simulink model "bObserver"  (R2020a)
settings: Solver=VariableStepAuto  StartTime=0.0  StopTime=1.5  FixedStep=0.0005  EnableMultiTasking=on
InitFcn:
  | kp=0.01;
  | ki=0.01;
  | 
  | k=2;
  | em=100000000;
  | GE=1/em;
  | GU=k*ki/GE;
  | GCE=k*kp/GU;
model workspace (MAT data in the model file):
  time = 0.8
values from neighbouring files (symbols this model uses):
  A1 = obj.boostConverter.A1    [BoostController.m]    (also in BoostConverter.m = [-obj.R/obj.L 0;0 -1/(obj.Ro*obj.C)]; BuckBoostConverter.m = [-obj.R/obj.L 0;0 -1/(obj.Ro*obj.C)]; obsmc.m = Asigma{1,1}; workspace_atual.mat = [-16.4  0; 0  -3.50877192982])
  A2 = obj.boostConverter.A2    [BoostController.m]    (also in BoostConverter.m = [-obj.R/obj.L -1/obj.L;1/obj.C -1/(obj.Ro*obj.C)]; BuckBoostConverter.m = [-obj.R/obj.L 1/obj.L;-1/obj.C -1/(obj.Ro*obj.C)]; obsmc.m = Asigma{1,2}; workspace_atual.mat = [-16.4  -200; 350.877192982  -3.50877192982])
  AlarmDeadTime = 0.50    (= 0.5)    [BoostFaultSimulation.m]    (also in workspace_atual.mat; workspace_certo.mat)
  B1 = obj.boostConverter.B1    [BoostController.m]    (also in BoostConverter.m = [1/obj.L;0]; BuckBoostConverter.m = [1/obj.L;0]; obsmc.m = Bsigma{1,1}; workspace_atual.mat = [200 0])
  B1f = [200 0]    [workspace_atual.mat]    (also in workspace_certo.mat)
  B2 = obj.boostConverter.B2    [BoostController.m]    (also in BoostConverter.m = obj.B1; obsmc.m = Bsigma{1,2}; workspace_atual.mat = [200 0]; workspace_certo.mat = [200 0])
  B2f = [200 0]    [workspace_atual.mat]    (also in workspace_certo.mat)
  boost_Amatrices = cat(3,obj.A1,obj.A2)    [BoostConverter.m]    (also in BuckBoostConverter.m; boostResults2Latex.m = boost.A_matrices(); workspace_atual.mat = [-16.4 0 0 -3.50877192982 -16.4 350.877192982 -200 -3.508771; workspace_certo.mat = [-16.4 0 0 -3.50877192982 -16.4 350.877192982 -200 -3.508771)
  boost_parameters = [obj.Ro,obj.R,obj.L,obj.C,obj.u]'    [BoostConverter.m]    (also in BuckBoostConverter.m; boostResults2Latex.m = boost.parameters(); workspace_atual.mat = [100 0.082 0.005 0.00285 190]; workspace_certo.mat = [100 0.082 0.005 0.00285 190])
  C = 1e-3    (= 0.001)    [boostResults2Latex.m]
  CiL = [0 1]    [workspace_atual.mat]    (also in workspace_certo.mat)
  Cmatrix = [1  0; 0  1]    [workspace_atual.mat]    (also in workspace_certo.mat)
  CVc = [1 0]    [workspace_atual.mat]    (also in workspace_certo.mat)
  D1 = [1  0; 0  1]    [workspace_atual.mat]    (also in workspace_certo.mat)
  F_11 = -16.4    [workspace_atual.mat]    (also in workspace_certo.mat)
  F_12 = -4812476.87956    [workspace_atual.mat]    (also in workspace_certo.mat)
  F_21 = -3.50877192982    [workspace_atual.mat]    (also in workspace_certo.mat)
  F_22 = -2.00703596657    [workspace_atual.mat]    (also in workspace_certo.mat)
  FaultClass = 0    [BoostFaultSimulation.m]    (also in workspace_atual.mat = 1; workspace_certo.mat = 1)
  H_1 = 13715.5123667    [workspace_atual.mat]    (also in workspace_certo.mat)
  iLFaultSwitch = 0    [BoostFaultSimulation.m]    (also in workspace_atual.mat; workspace_certo.mat)
  iLFaultTime = 1.70    (= 1.7)    [BoostFaultSimulation.m]    (also in workspace_atual.mat; workspace_certo.mat)
  iLGainFaultFactor = 15    [BoostFaultSimulation.m]    (also in workspace_atual.mat; workspace_certo.mat)
  iLNoiseFaultSwitch = 0    [BoostFaultSimulation.m]    (also in workspace_atual.mat; workspace_certo.mat)
  iLNoiseTime = 1.70    (= 1.7)    [BoostFaultSimulation.m]    (also in workspace_atual.mat; workspace_certo.mat)
  Jth = 2000    [workspace_atual.mat]    (also in workspace_certo.mat)
  L = 1e-3    (= 0.001)    [boostResults2Latex.m]    (also in obsmc.m = sdpvar(3,1,'full'))
  L_11 = -176809.798019    [workspace_atual.mat]    (also in workspace_certo.mat)
  L_12 = -66005538231.6    [workspace_atual.mat]    (also in workspace_certo.mat)
  L_21 = 0.0967961040176    [workspace_atual.mat]    (also in workspace_certo.mat)
  L_22 = 350.985265141    [workspace_atual.mat]    (also in workspace_certo.mat)
  LoadAddSignalSwitch = 1    [BoostFaultSimulation.m]    (also in workspace_atual.mat; workspace_certo.mat)
  LoadAddSwitch = 0    [BoostFaultSimulation.m]    (also in workspace_atual.mat; workspace_certo.mat)
  LoadAddTime = 0.90    (= 0.9)    [BoostFaultSimulation.m]    (also in workspace_atual.mat; workspace_certo.mat)
  LoadRemoveSignalSwitch = 1    [BoostFaultSimulation.m]    (also in workspace_atual.mat; workspace_certo.mat)
  LoadRemoveSwitch = 0    [BoostFaultSimulation.m]    (also in workspace_atual.mat; workspace_certo.mat)
  LoadRemoveTime = 0.90    (= 0.9)    [BoostFaultSimulation.m]    (also in workspace_atual.mat; workspace_certo.mat)
  LobsiL = [1737913.15707 66180.0912281]    [workspace_atual.mat]    (also in workspace_certo.mat)
  LobsVc = [61200 1]    [workspace_atual.mat]    (also in workspace_certo.mat)
  ObsEp = 70    [workspace_atual.mat]    (also in workspace_certo.mat)
  P = value(P)    [BoostController.m]    (also in boostResults2Latex.m = boost.calculateP(); obsmc.m = blkdiag(1/deltaAtilde(1,2),-1/deltaAtilde(2,1),1); workspace_atual.mat = [0.00235275094895  5.25738510027e-05; 5.25738510027e-05  0.0; workspace_certo.mat = [0.00235275094893  5.25738512446e-05; 5.25738512446e-05  0.0)
  Q_1 = [13715.5123667  1; 1  0]    [workspace_atual.mat]    (also in workspace_certo.mat)
  Q_2 = [1  0; 0.00750867981628  1]    [workspace_atual.mat]    (also in workspace_certo.mat)
  R = 0.1    [boostResults2Latex.m]    (also in workspace_atual.mat = 0.082; workspace_certo.mat = 0.082)
  ReconfigSwitch = 0    [BoostFaultSimulation.m]    (also in workspace_atual.mat; workspace_certo.mat)
  ReconfigTime = 1.707    [BoostFaultSimulation.m]    (also in workspace_atual.mat; workspace_certo.mat)
  rho = 5    [workspace_atual.mat]    (also in workspace_certo.mat)
  RMSfrequency = 47.61    [BoostFaultSimulation.m]    (also in workspace_atual.mat; workspace_certo.mat)
  Ro = 100    [BoostFaultSimulation.m]    (also in boostResults2Latex.m = 10; workspace_atual.mat; workspace_certo.mat)
  Smep = 80    [workspace_atual.mat]    (also in workspace_certo.mat)
  SourceAddSignalSwitch = 1    [BoostFaultSimulation.m]    (also in workspace_atual.mat; workspace_certo.mat)
  SourceAddSwitch = 0    [BoostFaultSimulation.m]    (also in workspace_atual.mat; workspace_certo.mat)
  SourceAddTime = 0.90    (= 0.9)    [BoostFaultSimulation.m]    (also in workspace_atual.mat; workspace_certo.mat)
  SourceAddVoltage = obj.SourceAddFactor*obj.u    [BoostFaultSimulation.m]    (also in workspace_atual.mat = 19; workspace_certo.mat = 19)
  SourceRemoveSignalSwitch = 1    [BoostFaultSimulation.m]    (also in workspace_atual.mat; workspace_certo.mat)
  SourceRemoveSwitch = 0    [BoostFaultSimulation.m]    (also in workspace_atual.mat; workspace_certo.mat)
  SourceRemoveTime = 0.90    (= 0.9)    [BoostFaultSimulation.m]    (also in workspace_atual.mat; workspace_certo.mat)
  SourceRemoveVoltage = obj.SourceRemoveFactor*obj.u    [BoostFaultSimulation.m]    (also in workspace_atual.mat = 19; workspace_certo.mat = 19)
  T_1 = [1 -13715.5123667]    [workspace_atual.mat]    (also in workspace_certo.mat)
  T_2 = [-0.00750867981628 1]    [workspace_atual.mat]    (also in workspace_certo.mat)
  ueq = 0.5    [workspace_atual.mat]    (also in workspace_certo.mat)
  uf = 190    [workspace_atual.mat]    (also in workspace_certo.mat)
  VcFaultSwitch = 0    [BoostFaultSimulation.m]    (also in workspace_atual.mat; workspace_certo.mat)
  VcFaultTime = 1.70    (= 1.7)    [BoostFaultSimulation.m]    (also in workspace_atual.mat; workspace_certo.mat)
  VcGainFaultFactor = 15    [BoostFaultSimulation.m]    (also in workspace_atual.mat; workspace_certo.mat)
  VcNoiseFaultSwitch = 0    [BoostFaultSimulation.m]    (also in workspace_atual.mat; workspace_certo.mat)
  VcNoiseTime = 1.70    (= 1.7)    [BoostFaultSimulation.m]    (also in workspace_atual.mat; workspace_certo.mat)
  ve = 380    [BoostFaultSimulation.m]    (also in boostResults2Latex.m = 100; workspace_atual.mat; workspace_certo.mat)
  x_e = [ie;ve]    [BoostConverter.m]    (also in BuckBoostConverter.m)
  xe = obj.boostConverter.equilibriumstate(ve)    [BoostController.m]    (also in workspace_atual.mat = [7.62509288104 380]; workspace_certo.mat = [7.62509288104 380])
undefined symbols (not defined in the file or in its folder): Atilde1, Atilde2, B1u, Ctilde1, Dtilde1, Dtilde2, F, F1, G, G1, MAXnet, MINnet
libraries: neural x36, powerlib x34, dspstat3 x11, PhdLibrary x10, simulink x7, dspmtrx3 x6, powerlib_meascontrol x4, dspmathops x4
(part 4 of 6)

== system bObserver/Slding Mode/ErrorGenerator/If Action Subsystem ==
  e_y : Inport
  Action Port : ActionPort  ActionPortLabel=if(u1 ~= 0)
  Matrix Multiply : Product  Multiplication=Matrix(*)
  Matrix Multiply1 : Product
  Matrizes A1 : Constant  Value=rho
  Matrizes A2 : Constant  Value=F
  Normalization : dspmathops/Normalization  NormType=2-norm  Bias=1e-10  NormOver=Each column  Dimension=1  roundingMode=Floor  overflowMode=off  accumDataTypeStr=Inherit: Same as product output  accumLastDataTypeStr=Inherit: Same as product output  outputDataTypeStr=Inherit: Same as product output  outputMin=[]  outputMax=[]  outputLastDataTypeStr=Inherit: Same as product output
  v : Outport
  wires:
  Matrix Multiply/1 -> Normalization/1
  Matrizes A2/1 -> Matrix Multiply/1
  Normalization/1 -> Matrix Multiply1/2
  e_y/1 -> Matrix Multiply/2
  Matrizes A1/1 -> Matrix Multiply1/1
  Matrix Multiply1/1 -> v/1

== system bObserver/Slding Mode/ErrorGenerator/If Action Subsystem1 ==
  e_y : Inport
  Action Port : ActionPort  ActionPortLabel=else
  v : Outport
  wires:
  e_y/1 -> v/1

== system bObserver/Slding Mode/Fault Identification Neural Netowrk/Pattern Recognition Neural Network1 ==
  Input : Inport  PortDimensions=3
      mask Display: e = 0.06;c1 = [120 230 180]/255;c2 = ([120 230 180]+0)/(256+128);c3 = ([120 230 180]+128)/(256+128);patch([0 1 1 0],[0 0 1 1],c1);patch([0 1 1 1-e 1-e 0+e],[0 0 1 1-e 0+e 0+e],c2);patch([0 0 1 1-e 0+e 0+e],[0 1 1 1-e 1-e 0+e],c3);plot([0 1 1 0 0],[0 0 1 1 0]);
  Layer 1 : Subsystem
      mask Display: e = 0.06;c1 = [120 150 230]/255;c2 = ([120 150 230]+0)/383;c3 = ([120 150 230]+128)/383;patch([0 1 1 0],[0 0 1 1],c1);patch([0 1 1 1-e 1-e 0+e],[0 0 1 1-e 0+e 0+e],c2);patch([0 0 1 1-e 0+e 0+e],[0 1 1 1-e 1-e 0+e],c3);plot([0 1 1 0 0],[0 0 1 1 0]);
  Layer 2 : Subsystem
      mask Display: e = 0.06;c1 = [120 150 230]/255;c2 = ([120 150 230]+0)/383;c3 = ([120 150 230]+128)/383;patch([0 1 1 0],[0 0 1 1],c1);patch([0 1 1 1-e 1-e 0+e],[0 0 1 1-e 0+e 0+e],c2);patch([0 0 1 1-e 0+e 0+e],[0 1 1 1-e 1-e 0+e],c3);plot([0 1 1 0 0],[0 0 1 1 0]);
  Process Input 1 : Subsystem
      mask Display: e = 0.06;c1 = [120 150 230]/255;c2 = ([120 150 230]+0)/383;c3 = ([120 150 230]+128)/383;patch([0 1 1 0],[0 0 1 1],c1);patch([0 1 1 1-e 1-e 0+e],[0 0 1 1-e 0+e 0+e],c2);patch([0 0 1 1-e 0+e 0+e],[0 1 1 1-e 1-e 0+e],c3);plot([0 1 1 0 0],[0 0 1 1 0]);
  Process Output 1 : Subsystem
      mask Display: e = 0.06;c1 = [120 150 230]/255;c2 = ([120 150 230]+0)/383;c3 = ([120 150 230]+128)/383;patch([0 1 1 0],[0 0 1 1],c1);patch([0 1 1 1-e 1-e 0+e],[0 0 1 1-e 0+e 0+e],c2);patch([0 0 1 1-e 0+e 0+e],[0 1 1 1-e 1-e 0+e],c3);plot([0 1 1 0 0],[0 0 1 1 0]);
  Output : Outport  InitialOutput=[0;0;0;0;0]
      mask Display: e = 0.06;c1 = [120 230 180]/255;c2 = ([120 230 180]+0)/(256+128);c3 = ([120 230 180]+128)/(256+128);patch([0 1 1 0],[0 0 1 1],c1);patch([0 1 1 1-e 1-e 0+e],[0 0 1 1-e 0+e 0+e],c2);patch([0 0 1 1-e 0+e 0+e],[0 1 1 1-e 1-e 0+e],c3);plot([0 1 1 0 0],[0 0 1 1 0]);
  wires:
  Input/1 -> Process Input 1/1(x)
  Process Output 1/1(y) -> Output/1
  Process Input 1/1(p) -> Layer 1/1("p{1}")
  Layer 1/1("a{1}") -> [feedback1]
  [feedback1] -> Layer 2/1("a{1} ")
  Layer 2/1("a{2}") -> Process Output 1/1(a)

== system bObserver/Slding Mode/Fault Identification Neural Netowrk/Subsystem ==
  input : Inport
  min : Inport  Port=2
  max : Inport  Port=3
  Constant2 : Constant  Value=2
  Constant3 : Constant
  Divide : Product  Inputs=*/
  Product : Product
  Sum : Sum  Inputs=|+-
  Sum1 : Sum  Inputs=|+-
  Sum2 : Sum  Inputs=|+-
  Out1 : Outport
  wires:
  Divide/1 -> Product/2
  max/1 -> Sum2/1
  Constant3/1 -> Sum1/2
  Product/1 -> Sum1/1
  input/1 -> Sum/1
  Sum/1 -> Divide/1
  Sum2/1 -> Divide/2
  Constant2/1 -> Product/1
  Sum1/1 -> Out1/1
  min/1 -> Sum/2, Sum2/2

== system bObserver/Slding Mode/Fault Identification Neural Netowrk/Subsystem1 ==
  input : Inport
  min : Inport  Port=2
  max : Inport  Port=3
  Constant2 : Constant  Value=2
  Constant3 : Constant
  Divide : Product  Inputs=*/
  Product : Product
  Sum : Sum  Inputs=|+-
  Sum1 : Sum  Inputs=|+-
  Sum2 : Sum  Inputs=|+-
  Out1 : Outport
  wires:
  Divide/1 -> Product/2
  max/1 -> Sum2/1
  Constant3/1 -> Sum1/2
  Product/1 -> Sum1/1
  input/1 -> Sum/1
  Sum/1 -> Divide/1
  Sum2/1 -> Divide/2
  Constant2/1 -> Product/1
  Sum1/1 -> Out1/1
  min/1 -> Sum/2, Sum2/2

== system bObserver/Slding Mode/Fault Identification Neural Netowrk/Subsystem2 ==
  input : Inport
  min : Inport  Port=2
  max : Inport  Port=3
  Constant2 : Constant  Value=2
  Constant3 : Constant
  Divide : Product  Inputs=*/
  Product : Product
  Sum : Sum  Inputs=|+-
  Sum1 : Sum  Inputs=|+-
  Sum2 : Sum  Inputs=|+-
  Out1 : Outport
  wires:
  Divide/1 -> Product/2
  max/1 -> Sum2/1
  Constant3/1 -> Sum1/2
  Product/1 -> Sum1/1
  input/1 -> Sum/1
  Sum/1 -> Divide/1
  Sum2/1 -> Divide/2
  Constant2/1 -> Product/1
  Sum1/1 -> Out1/1
  min/1 -> Sum/2, Sum2/2

== system bObserver/Slding Mode/Sliding Mode Observer 5/ObserverDynamics ==
  ey : Inport
  v : Inport  Port=2
  sigma : Inport  Port=3
  Gain : Gain  Gain=Atilde1  Multiplication=Matrix(K*u)
  Gain1 : Gain  Gain=G  Multiplication=Matrix(K*u)
  Gain3 : Gain  Gain=Dtilde1  Multiplication=Matrix(K*u)
  Gain5 : Gain  Gain=Atilde2  Multiplication=Matrix(K*u)
  Gain7 : Gain  Gain=Dtilde2  Multiplication=Matrix(K*u)
  Integral : Subsystem
  Sum : Sum  Inputs=|+++
  Sum1 : Sum  Inputs=|+++
  Switch1 : Switch  Criteria=u2 > Threshold
  e_tilde_hat : Outport
  wires:
  sigma/1 -> Switch1/2
  Switch1/1 -> Integral/1(e_hat_dot)  "v"
  Integral/1(e_hat) -> Gain/1, e_tilde_hat/1, Gain5/1
  ey/1 -> Gain1/1
  v/1 -> Gain7/1, Gain3/1
  Sum1/1 -> Switch1/3
  Sum/1 -> Switch1/1
  Gain7/1 -> Sum1/2
  Gain5/1 -> Sum1/3
  Gain3/1 -> Sum/1
  Gain1/1 -> Sum1/1, Sum/2
  Gain/1 -> Sum/3

== system bObserver/Slding Mode/Subsystem/SlidingSurface ==
  S : Inport
  ep : Inport  Port=2
  Abs : Abs  ZeroCross=off
  GreaterThan : RelationalOperator  Operator=>  OutDataTypeStr=boolean  RndMeth=Simplest
  If : If  IfExpression=u1 ~= 0
  If Action Subsystem : Subsystem  TreatAsAtomicUnit=on
  If Action Subsystem2 : Subsystem  TreatAsAtomicUnit=on
  Merge1 : Merge
  d : Outport
  wires:
  If Action Subsystem2/1(d) -> Merge1/2
  [S] -> If Action Subsystem/1(S), If Action Subsystem2/1(S)
  If/2 -> If Action Subsystem2/Action
  If/1 -> If Action Subsystem/Action
  [ep] -> If Action Subsystem2/2(ep)
  S/1 -> [S], Abs/1
  If Action Subsystem/1(d) -> Merge1/1
  Abs/1 -> GreaterThan/1
  GreaterThan/1 -> If/1
  Merge1/1 -> d/1
  ep/1 -> [ep], GreaterThan/2

== system bObserver/Slding Mode/Subsystem1/SlidingSurface ==
  S : Inport
  ep : Inport  Port=2
  Abs : Abs  ZeroCross=off
  GreaterThan : RelationalOperator  Operator=>  OutDataTypeStr=boolean  RndMeth=Simplest
  If : If  IfExpression=u1 ~= 0
  If Action Subsystem : Subsystem  TreatAsAtomicUnit=on
  If Action Subsystem2 : Subsystem  TreatAsAtomicUnit=on
  Merge1 : Merge
  d : Outport
  wires:
  If Action Subsystem2/1(d) -> Merge1/2
  [S] -> If Action Subsystem/1(S), If Action Subsystem2/1(S)
  If/2 -> If Action Subsystem2/Action
  If/1 -> If Action Subsystem/Action
  [ep] -> If Action Subsystem2/2(ep)
  S/1 -> [S], Abs/1
  If Action Subsystem/1(d) -> Merge1/1
  Abs/1 -> GreaterThan/1
  GreaterThan/1 -> If/1
  Merge1/1 -> d/1
  ep/1 -> [ep], GreaterThan/2

== system bObserver/Slding Mode/Subsystem9/Residual Generator2 ==
  e_y : Inport
  Matrix Square1 : dspmtrx3/Matrix Square  OutMin=[]  OutMax=[]
      settings: SourceProductBaseCode=DS
  Moving RMS : dspstat3/Moving RMS  Method=Sliding window  ForgettingFactorPort=off  SpecifyWindowLength=on  WindowLength=RMSfrequency/10  ForgettingFactor=0.9  SimulateUsing=Code generation
      settings: SourceProductBaseCode=DS
  Sqrt2 : Sqrt  SaturateOnIntegerOverflow=on
  RMS : Outport
  wires:
  Matrix Square1/1 -> Sqrt2/1
  e_y/1 -> Matrix Square1/1
  Sqrt2/1 -> Moving RMS/1
  Moving RMS/1 -> RMS/1

== system bObserver/Slding Mode/Vc OBserver/calc_x_hat ==
  sigma : Inport
  rsign : Inport  Port=2
  Lobs : Inport  Port=3
  Gain : Gain  Gain=A1  Multiplication=Matrix(K*u)
  Gain5 : Gain  Gain=A2  Multiplication=Matrix(K*u)
  Integral : Subsystem
  Matrix Multiply : Product  Multiplication=Matrix(*)
  MatrizesA8 : Constant  Value=B1*u
  Scope1 : Scope
  Sum : Sum  Inputs=|+++
  Sum1 : Sum  Inputs=|+++
  Switch1 : Switch  Criteria=u2 ~= 0
  x_hat : Outport
  wires:
  sigma/1 -> Switch1/2
  Switch1/1 -> Integral/1(x_hat_dot)  "v"
  Integral/1(x_hat) -> Scope1/1, x_hat/1, Gain/1, Gain5/1
  Sum1/1 -> Switch1/3
  Sum/1 -> Switch1/1
  Gain/1 -> Sum/3
  Gain5/1 -> Sum1/3
  Matrix Multiply/1 -> Sum/2, Sum1/2
  MatrizesA8/1 -> Sum1/1, Sum/1
  Lobs/1 -> Matrix Multiply/1
  rsign/1 -> Matrix Multiply/2

== system bObserver/Slding Mode/iL Observer/calc_x_hat ==
  sigma : Inport
  rsign : Inport  Port=2
  Lobs : Inport  Port=3
  Gain : Gain  Gain=A1  Multiplication=Matrix(K*u)
  Gain5 : Gain  Gain=A2  Multiplication=Matrix(K*u)
  Integral : Subsystem
  Matrix Multiply : Product  Multiplication=Matrix(*)
  MatrizesA8 : Constant  Value=B1*u
  Scope1 : Scope
  Sum : Sum  Inputs=|+++
  Sum1 : Sum  Inputs=|+++
  Switch1 : Switch  Criteria=u2 ~= 0
  x_hat : Outport
  wires:
  sigma/1 -> Switch1/2
  Switch1/1 -> Integral/1(x_hat_dot)  "v"
  Integral/1(x_hat) -> Scope1/1, x_hat/1, Gain/1, Gain5/1
  Sum1/1 -> Switch1/3
  Sum/1 -> Switch1/1
  Gain/1 -> Sum/3
  Gain5/1 -> Sum1/3
  Matrix Multiply/1 -> Sum/2, Sum1/2
  MatrizesA8/1 -> Sum1/1, Sum/1
  Lobs/1 -> Matrix Multiply/1
  rsign/1 -> Matrix Multiply/2

== system bObserver/ROSLSO/Bank of ROSLSO/z1/Integral ==
  z_dot : Inport
  Ground : Ground
  IC : InitialCondition  Value=0
  Integrator1 : Integrator  InitialConditionSource=external  InitialCondition=[-x_e; 0; 0]
  z : Outport
  wires:
  z_dot/1 -> Integrator1/1
  Integrator1/1 -> z/1
  Ground/1 -> IC/1
  IC/1 -> Integrator1/2

== system bObserver/ROSLSO/Bank of ROSLSO/z3/Integral ==
  z_dot : Inport
  Ground : Ground
  IC : InitialCondition  Value=0
  Integrator1 : Integrator  InitialConditionSource=external  InitialCondition=[-x_e; 0; 0]
  z : Outport
  wires:
  z_dot/1 -> Integrator1/1
  Integrator1/1 -> z/1
  Ground/1 -> IC/1
  IC/1 -> Integrator1/2

== system bObserver/ROSLSO/Bank of ROSLSO/z4/Integral ==
  z_dot : Inport
  Ground : Ground
  IC : InitialCondition  Value=0
  Integrator1 : Integrator  InitialConditionSource=external  InitialCondition=[-x_e; 0; 0]
  z : Outport
  wires:
  z_dot/1 -> Integrator1/1
  Integrator1/1 -> z/1
  Ground/1 -> IC/1
  IC/1 -> Integrator1/2

== system bObserver/ROSLSO/Bank of ROSMO/Subsystem/SlidingSurface ==
  S : Inport
  ep : Inport  Port=2
  Abs : Abs  ZeroCross=off
  GreaterThan : RelationalOperator  Operator=>  OutDataTypeStr=boolean  RndMeth=Simplest
  If : If  IfExpression=u1 ~= 0
  If Action Subsystem : Subsystem  TreatAsAtomicUnit=on
  If Action Subsystem2 : Subsystem  TreatAsAtomicUnit=on
  Merge1 : Merge
  d : Outport
  wires:
  If Action Subsystem2/1(d) -> Merge1/2
  [S] -> If Action Subsystem/1(S), If Action Subsystem2/1(S)
  If/2 -> If Action Subsystem2/Action
  If/1 -> If Action Subsystem/Action
  [ep] -> If Action Subsystem2/2(ep)
  S/1 -> [S], Abs/1
  If Action Subsystem/1(d) -> Merge1/1
  Abs/1 -> GreaterThan/1
  GreaterThan/1 -> If/1
  Merge1/1 -> d/1
  ep/1 -> [ep], GreaterThan/2

== system bObserver/ROSLSO/Bank of ROSMO/Subsystem1/SlidingSurface ==
  S : Inport
  ep : Inport  Port=2
  Abs : Abs  ZeroCross=off
  GreaterThan : RelationalOperator  Operator=>  OutDataTypeStr=boolean  RndMeth=Simplest
  If : If  IfExpression=u1 ~= 0
  If Action Subsystem : Subsystem  TreatAsAtomicUnit=on
  If Action Subsystem2 : Subsystem  TreatAsAtomicUnit=on
  Merge1 : Merge
  d : Outport
  wires:
  If Action Subsystem2/1(d) -> Merge1/2
  [S] -> If Action Subsystem/1(S), If Action Subsystem2/1(S)
  If/2 -> If Action Subsystem2/Action
  If/1 -> If Action Subsystem/Action
  [ep] -> If Action Subsystem2/2(ep)
  S/1 -> [S], Abs/1
  If Action Subsystem/1(d) -> Merge1/1
  Abs/1 -> GreaterThan/1
  GreaterThan/1 -> If/1
  Merge1/1 -> d/1
  ep/1 -> [ep], GreaterThan/2

== system bObserver/ROSLSO/Bank of ROSMO/Vc OBserver/calc_x_hat ==
  sigma : Inport
  rsign : Inport  Port=2
  Lobs : Inport  Port=3
  Gain : Gain  Gain=A1  Multiplication=Matrix(K*u)
  Gain5 : Gain  Gain=A2  Multiplication=Matrix(K*u)
  Integral : Subsystem
  Matrix Multiply : Product  Multiplication=Matrix(*)
  MatrizesA8 : Constant  Value=B1*u
  Scope1 : Scope
  Sum : Sum  Inputs=|+++
  Sum1 : Sum  Inputs=|+++
  Switch1 : Switch  Criteria=u2 ~= 0
  x_hat : Outport
  wires:
  sigma/1 -> Switch1/2
  Switch1/1 -> Integral/1(x_hat_dot)  "v"
  Integral/1(x_hat) -> Scope1/1, x_hat/1, Gain/1, Gain5/1
  Sum1/1 -> Switch1/3
  Sum/1 -> Switch1/1
  Gain/1 -> Sum/3
  Gain5/1 -> Sum1/3
  Matrix Multiply/1 -> Sum/2, Sum1/2
  MatrizesA8/1 -> Sum1/1, Sum/1
  Lobs/1 -> Matrix Multiply/1
  rsign/1 -> Matrix Multiply/2

== system bObserver/ROSLSO/Bank of ROSMO/iL Observer/calc_x_hat ==
  sigma : Inport
  rsign : Inport  Port=2
  Lobs : Inport  Port=3
  Gain : Gain  Gain=A1  Multiplication=Matrix(K*u)
  Gain5 : Gain  Gain=A2  Multiplication=Matrix(K*u)
  Integral : Subsystem
  Matrix Multiply : Product  Multiplication=Matrix(*)
  MatrizesA8 : Constant  Value=B1*u
  Scope1 : Scope
  Sum : Sum  Inputs=|+++
  Sum1 : Sum  Inputs=|+++
  Switch1 : Switch  Criteria=u2 ~= 0
  x_hat : Outport
  wires:
  sigma/1 -> Switch1/2
  Switch1/1 -> Integral/1(x_hat_dot)  "v"
  Integral/1(x_hat) -> Scope1/1, x_hat/1, Gain/1, Gain5/1
  Sum1/1 -> Switch1/3
  Sum/1 -> Switch1/1
  Gain/1 -> Sum/3
  Gain5/1 -> Sum1/3
  Matrix Multiply/1 -> Sum/2, Sum1/2
  MatrizesA8/1 -> Sum1/1, Sum/1
  Lobs/1 -> Matrix Multiply/1
  rsign/1 -> Matrix Multiply/2

== system bObserver/ROSLSO/Chaveado_fixo1/Controlador Chavead/MatirxControle ==
  "boost_parameters " : Inport
  boost_Amatrices : Inport  Port=2
  P : Inport  Port=3
  ve : Inport  Port=4
  x : Inport  Port=5
  To Workspace : ToWorkspace  VariableName=control_matrix2  SampleTime=-1
  "control_law " : MATLAB Function  TreatAsAtomicUnit=on
  xe : MATLAB Function  TreatAsAtomicUnit=on
  sigma : Outport
  x_e : Outport  Port=2
  i_e : Outport  Port=3
  wires:
  "control_law "/2(control_matrix) -> To Workspace/1
  "boost_parameters "/1 -> xe/1(boost_parameters)
  ve/1 -> xe/2(ve)
  P/1 -> "control_law "/2(P)
  boost_Amatrices/1 -> "control_law "/3(boost_Amatrices)
  "control_law "/1(sigma) -> sigma/1
  x/1 -> "control_law "/4(x)
  xe/2(x_e) -> x_e/1, "control_law "/1(x_e)
  xe/1(i_e) -> i_e/1

== system bObserver/ROSLSO/Controlador1/SlidingSurface/If Action Subsystem ==
  S : Inport
  Action Port : ActionPort  ActionPortLabel=if(u1 ~= 0)
  Sign : Signum
  d : Outport
  wires:
  S/1 -> Sign/1
  Sign/1 -> d/1

== system bObserver/ROSLSO/Controlador1/SlidingSurface/If Action Subsystem2 ==
  S : Inport
  ep : Inport  Port=2
  Action Port : ActionPort  ActionPortLabel=else
  Divide : Product  Inputs=*/
  d : Outport
  wires:
  S/1 -> Divide/1
  ep/1 -> Divide/2
  Divide/1 -> d/1

== system bObserver/ROSLSO/Fault Diagnostics/Augmented Error Generator/z1 ==
  z_dot : Inport
  Constant1 : Constant  Value=[0;0]  VectorParams1D=off
  Gain2 : Gain  Gain=Cmatrix  Multiplication=Matrix(K*u) (u vector)
  Integrator6 : Integrator  InitialConditionSource=external
  z : Outport
  wires:
  Gain2/1 -> Integrator6/1
  Integrator6/1 -> z/1
  z_dot/1 -> Gain2/1
  Constant1/1 -> Integrator6/2

== system bObserver/ROSLSO/Fault Diagnostics/ErrorGenerator/If Action Subsystem ==
  e_y : Inport
  Action Port : ActionPort
  Matrix Multiply : Product  Multiplication=Matrix(*)
  Matrix Multiply1 : Product
  Matrizes A1 : Constant  Value=rho
  Matrizes A2 : Constant  Value=F
  Normalization : dspmathops/Normalization  NormType=2-norm  Bias=1e-10  NormOver=Each column  Dimension=1  roundingMode=Floor  overflowMode=off  accumDataTypeStr=Inherit: Same as product output  accumLastDataTypeStr=Inherit: Same as product output  outputDataTypeStr=Inherit: Same as product output  outputMin=[]  outputMax=[]  outputLastDataTypeStr=Inherit: Same as product output
  v : Outport
  wires:
  Matrix Multiply/1 -> Normalization/1
  Matrizes A2/1 -> Matrix Multiply/1
  Normalization/1 -> Matrix Multiply1/2
  e_y/1 -> Matrix Multiply/2
  Matrizes A1/1 -> Matrix Multiply1/1
  Matrix Multiply1/1 -> v/1

== system bObserver/ROSLSO/Fault Diagnostics/ErrorGenerator/If Action Subsystem1 ==
  e_y : Inport
  Action Port : ActionPort
  v : Outport
  wires:
  e_y/1 -> v/1

== system bObserver/ROSLSO/Fault Diagnostics/Fault Identification Neural Netowrk/Pattern Recognition Neural Network1 ==
  Input : Inport  PortDimensions=3
      mask Display: e = 0.06;c1 = [120 230 180]/255;c2 = ([120 230 180]+0)/(256+128);c3 = ([120 230 180]+128)/(256+128);patch([0 1 1 0],[0 0 1 1],c1);patch([0 1 1 1-e 1-e 0+e],[0 0 1 1-e 0+e 0+e],c2);patch([0 0 1 1-e 0+e 0+e],[0 1 1 1-e 1-e 0+e],c3);plot([0 1 1 0 0],[0 0 1 1 0]);
  Layer 1 : Subsystem
      mask Display: e = 0.06;c1 = [120 150 230]/255;c2 = ([120 150 230]+0)/383;c3 = ([120 150 230]+128)/383;patch([0 1 1 0],[0 0 1 1],c1);patch([0 1 1 1-e 1-e 0+e],[0 0 1 1-e 0+e 0+e],c2);patch([0 0 1 1-e 0+e 0+e],[0 1 1 1-e 1-e 0+e],c3);plot([0 1 1 0 0],[0 0 1 1 0]);
  Layer 2 : Subsystem
      mask Display: e = 0.06;c1 = [120 150 230]/255;c2 = ([120 150 230]+0)/383;c3 = ([120 150 230]+128)/383;patch([0 1 1 0],[0 0 1 1],c1);patch([0 1 1 1-e 1-e 0+e],[0 0 1 1-e 0+e 0+e],c2);patch([0 0 1 1-e 0+e 0+e],[0 1 1 1-e 1-e 0+e],c3);plot([0 1 1 0 0],[0 0 1 1 0]);
  Process Input 1 : Subsystem
      mask Display: e = 0.06;c1 = [120 150 230]/255;c2 = ([120 150 230]+0)/383;c3 = ([120 150 230]+128)/383;patch([0 1 1 0],[0 0 1 1],c1);patch([0 1 1 1-e 1-e 0+e],[0 0 1 1-e 0+e 0+e],c2);patch([0 0 1 1-e 0+e 0+e],[0 1 1 1-e 1-e 0+e],c3);plot([0 1 1 0 0],[0 0 1 1 0]);
  Process Output 1 : Subsystem
      mask Display: e = 0.06;c1 = [120 150 230]/255;c2 = ([120 150 230]+0)/383;c3 = ([120 150 230]+128)/383;patch([0 1 1 0],[0 0 1 1],c1);patch([0 1 1 1-e 1-e 0+e],[0 0 1 1-e 0+e 0+e],c2);patch([0 0 1 1-e 0+e 0+e],[0 1 1 1-e 1-e 0+e],c3);plot([0 1 1 0 0],[0 0 1 1 0]);
  Output : Outport  InitialOutput=[0;0;0;0;0]
      mask Display: e = 0.06;c1 = [120 230 180]/255;c2 = ([120 230 180]+0)/(256+128);c3 = ([120 230 180]+128)/(256+128);patch([0 1 1 0],[0 0 1 1],c1);patch([0 1 1 1-e 1-e 0+e],[0 0 1 1-e 0+e 0+e],c2);patch([0 0 1 1-e 0+e 0+e],[0 1 1 1-e 1-e 0+e],c3);plot([0 1 1 0 0],[0 0 1 1 0]);
  wires:
  Input/1 -> Process Input 1/1(x)
  Process Output 1/1(y) -> Output/1
  Process Input 1/1(p) -> Layer 1/1("p{1}")
  Layer 1/1("a{1}") -> [feedback1]
  [feedback1] -> Layer 2/1("a{1} ")
  Layer 2/1("a{2}") -> Process Output 1/1(a)

== system bObserver/ROSLSO/Fault Diagnostics/Fault Identification Neural Netowrk/Subsystem ==
  input : Inport
  min : Inport  Port=2
  max : Inport  Port=3
  Constant2 : Constant  Value=2
  Constant3 : Constant
  Divide : Product  Inputs=*/
  Product : Product
  Sum : Sum  Inputs=|+-
  Sum1 : Sum  Inputs=|+-
  Sum2 : Sum  Inputs=|+-
  Out1 : Outport
  wires:
  Divide/1 -> Product/2
  max/1 -> Sum2/1
  Constant3/1 -> Sum1/2
  Product/1 -> Sum1/1
  input/1 -> Sum/1
  Sum/1 -> Divide/1
  Sum2/1 -> Divide/2
  Constant2/1 -> Product/1
  Sum1/1 -> Out1/1
  min/1 -> Sum/2, Sum2/2

== system bObserver/ROSLSO/Fault Diagnostics/Fault Identification Neural Netowrk/Subsystem1 ==
  input : Inport
  min : Inport  Port=2
  max : Inport  Port=3
  Constant2 : Constant  Value=2
  Constant3 : Constant
  Divide : Product  Inputs=*/
  Product : Product
  Sum : Sum  Inputs=|+-
  Sum1 : Sum  Inputs=|+-
  Sum2 : Sum  Inputs=|+-
  Out1 : Outport
  wires:
  Divide/1 -> Product/2
  max/1 -> Sum2/1
  Constant3/1 -> Sum1/2
  Product/1 -> Sum1/1
  input/1 -> Sum/1
  Sum/1 -> Divide/1
  Sum2/1 -> Divide/2
  Constant2/1 -> Product/1
  Sum1/1 -> Out1/1
  min/1 -> Sum/2, Sum2/2

== system bObserver/ROSLSO/Fault Diagnostics/Fault Identification Neural Netowrk/Subsystem2 ==
  input : Inport
  min : Inport  Port=2
  max : Inport  Port=3
  Constant2 : Constant  Value=2
  Constant3 : Constant
  Divide : Product  Inputs=*/
  Product : Product
  Sum : Sum  Inputs=|+-
  Sum1 : Sum  Inputs=|+-
  Sum2 : Sum  Inputs=|+-
  Out1 : Outport
  wires:
  Divide/1 -> Product/2
  max/1 -> Sum2/1
  Constant3/1 -> Sum1/2
  Product/1 -> Sum1/1
  input/1 -> Sum/1
  Sum/1 -> Divide/1
  Sum2/1 -> Divide/2
  Constant2/1 -> Product/1
  Sum1/1 -> Out1/1
  min/1 -> Sum/2, Sum2/2

== system bObserver/ROSLSO/Fault Diagnostics/Sliding Mode Observer 5/ObserverDynamics ==
  ey : Inport
  v : Inport  Port=2
  sigma : Inport  Port=3
  Gain : Gain  Gain=Atilde1  Multiplication=Matrix(K*u)
  Gain1 : Gain  Gain=G  Multiplication=Matrix(K*u)
  Gain3 : Gain  Gain=Dtilde1  Multiplication=Matrix(K*u)
  Gain5 : Gain  Gain=Atilde2  Multiplication=Matrix(K*u)
  Gain7 : Gain  Gain=Dtilde2  Multiplication=Matrix(K*u)
  Integral : Subsystem
  Sum : Sum  Inputs=|+++
  Sum1 : Sum  Inputs=|+++
  Switch1 : Switch  Criteria=u2 > Threshold
  e_tilde_hat : Outport
  wires:
  sigma/1 -> Switch1/2
  Switch1/1 -> Integral/1(e_hat_dot)  "v"
  Integral/1(e_hat) -> Gain/1, e_tilde_hat/1, Gain5/1
  ey/1 -> Gain1/1
  v/1 -> Gain7/1, Gain3/1
  Sum1/1 -> Switch1/3
  Sum/1 -> Switch1/1
  Gain7/1 -> Sum1/2
  Gain5/1 -> Sum1/3
  Gain3/1 -> Sum/1
  Gain1/1 -> Sum1/1, Sum/2
  Gain/1 -> Sum/3

== system bObserver/ROSLSO/Fault Diagnostics/Subsystem9/Residual Generator2 ==
  e_y : Inport
  Matrix Square1 : dspmtrx3/Matrix Square  OutMin=[]  OutMax=[]
      settings: SourceProductBaseCode=DS
  Moving RMS : dspstat3/Moving RMS  Method=Sliding window  ForgettingFactorPort=off  SpecifyWindowLength=on  WindowLength=RMSfrequency/10  ForgettingFactor=0.9  SimulateUsing=Code generation
      settings: SourceProductBaseCode=DS
  Sqrt2 : Sqrt  SaturateOnIntegerOverflow=on
  RMS : Outport
  wires:
  Matrix Square1/1 -> Sqrt2/1
  e_y/1 -> Matrix Square1/1
  Sqrt2/1 -> Moving RMS/1
  Moving RMS/1 -> RMS/1

== system bObserver/ROSMO_L1/Controlador2/SlidingSurface/If Action Subsystem ==
  S : Inport
  Action Port : ActionPort  ActionPortLabel=if(u1 ~= 0)
  Sign : Signum
  d : Outport
  wires:
  S/1 -> Sign/1
  Sign/1 -> d/1

== system bObserver/ROSMO_L1/Controlador2/SlidingSurface/If Action Subsystem2 ==
  S : Inport
  ep : Inport  Port=2
  Action Port : ActionPort  ActionPortLabel=else
  Divide : Product  Inputs=*/
  d : Outport
  wires:
  S/1 -> Divide/1
  ep/1 -> Divide/2
  Divide/1 -> d/1

== system bObserver/ROSMO_L1/SMO/ErrorGenerator/If Action Subsystem ==
  e_y : Inport
  Action Port : ActionPort  ActionPortLabel=if(u1 ~= 0)
  Matrix Multiply : Product  Multiplication=Matrix(*)
  Matrix Multiply1 : Product
  Matrizes A1 : Constant  Value=rho
  Matrizes A2 : Constant  Value=F  VectorParams1D=off
  Normalization : dspmathops/Normalization  NormType=2-norm  Bias=1e-10  NormOver=Each column  Dimension=1  roundingMode=Floor  overflowMode=off  accumDataTypeStr=Inherit: Same as product output  accumLastDataTypeStr=Inherit: Same as product output  outputDataTypeStr=Inherit: Same as product output  outputMin=[]  outputMax=[]  outputLastDataTypeStr=Inherit: Same as product output
  v : Outport
  wires:
  Matrix Multiply/1 -> Normalization/1
  Matrizes A2/1 -> Matrix Multiply/1
  Normalization/1 -> Matrix Multiply1/2
  e_y/1 -> Matrix Multiply/2
  Matrizes A1/1 -> Matrix Multiply1/1
  Matrix Multiply1/1 -> v/1

== system bObserver/ROSMO_L1/SMO/ErrorGenerator/If Action Subsystem1 ==
  e_y : Inport
  Action Port : ActionPort  ActionPortLabel=else
  v : Outport
  wires:
  e_y/1 -> v/1

== system bObserver/ROSMO_L1/SMO/Sliding Mode Observer 5/ObserverDynamics ==
  ey : Inport
  v : Inport  Port=2
  sigma : Inport  Port=3
  Gain : Gain  Gain=Atilde1  Multiplication=Matrix(K*u)
  Gain1 : Gain  Gain=G  Multiplication=Matrix(K*u)
  Gain3 : Gain  Gain=Dtilde1  Multiplication=Matrix(K*u)
  Gain5 : Gain  Gain=Atilde2  Multiplication=Matrix(K*u)
  Gain7 : Gain  Gain=Dtilde2  Multiplication=Matrix(K*u)
  Integral : Subsystem
  Sum : Sum  Inputs=|+++
  Sum1 : Sum  Inputs=|+++
  Switch1 : Switch  Criteria=u2 > Threshold
  e_tilde_hat : Outport
  wires:
  sigma/1 -> Switch1/2
  Switch1/1 -> Integral/1(e_hat_dot)  "v"
  Integral/1(e_hat) -> Gain/1, e_tilde_hat/1, Gain5/1
  ey/1 -> Gain1/1
  v/1 -> Gain7/1, Gain3/1
  Sum1/1 -> Switch1/3
  Sum/1 -> Switch1/1
  Gain7/1 -> Sum1/2
  Gain5/1 -> Sum1/3
  Gain3/1 -> Sum/1
  Gain1/1 -> Sum1/1, Sum/2
  Gain/1 -> Sum/3

== system bObserver/ROSMO_ROSLSO/Bank of ROSLSO/ROSLSO 2 Subsystems/Reduced Order Derivate Z ==
  u : Inport
  y : Inport  Port=2
  z : Inport  Port=3
  Constant : Constant  Value=F  VectorParams1D=off
  Constant1 : Constant  Value=T  VectorParams1D=off
  Constant2 : Constant  Value=L  VectorParams1D=off
  Matrix Multiply{1..3,8} (4 alike) : Product  Multiplication=Matrix(*)
  MatrizesA8 : Constant  Value=B  VectorParams1D=off
  Sum : Sum  Inputs=|+++
  zdot : Outport
  wires:
  MatrizesA8/1 -> Matrix Multiply8/1
  Constant1/1 -> Matrix Multiply1/1
  z/1 -> Matrix Multiply3/2
  Matrix Multiply3/1 -> Sum/2
  Constant/1 -> Matrix Multiply3/1
  Matrix Multiply8/1 -> Matrix Multiply1/2
  Matrix Multiply1/1 -> Sum/1
  u/1 -> Matrix Multiply8/2
  Sum/1 -> zdot/1
  Constant2/1 -> Matrix Multiply2/1
  Matrix Multiply2/1 -> Sum/3
  y/1 -> Matrix Multiply2/2

== system bObserver/ROSMO_ROSLSO/Bank of ROSLSO/ROSLSO 2 Subsystems/Reduced Order Derivate Z1 ==
  u : Inport
  y : Inport  Port=2
  z : Inport  Port=3
  Constant : Constant  Value=F  VectorParams1D=off
  Constant1 : Constant  Value=T  VectorParams1D=off
  Constant2 : Constant  Value=L  VectorParams1D=off
  Matrix Multiply{1..3,8} (4 alike) : Product  Multiplication=Matrix(*)
  MatrizesA8 : Constant  Value=B  VectorParams1D=off
  Sum : Sum  Inputs=|+++
  zdot : Outport
  wires:
  MatrizesA8/1 -> Matrix Multiply8/1
  Constant1/1 -> Matrix Multiply1/1
  z/1 -> Matrix Multiply3/2
  Matrix Multiply3/1 -> Sum/2
  Constant/1 -> Matrix Multiply3/1
  Matrix Multiply8/1 -> Matrix Multiply1/2
  Matrix Multiply1/1 -> Sum/1
  u/1 -> Matrix Multiply8/2
  Sum/1 -> zdot/1
  Constant2/1 -> Matrix Multiply2/1
  Matrix Multiply2/1 -> Sum/3
  y/1 -> Matrix Multiply2/2

== system bObserver/ROSMO_ROSLSO/Bank of ROSLSO/ROSLSO 2 Subsystems1/Reduced Order Derivate Z ==
  u : Inport
  y : Inport  Port=2
  z : Inport  Port=3
  Constant : Constant  Value=F  VectorParams1D=off
  Constant1 : Constant  Value=T  VectorParams1D=off
  Constant2 : Constant  Value=L  VectorParams1D=off
  Matrix Multiply{1..3,8} (4 alike) : Product  Multiplication=Matrix(*)
  MatrizesA8 : Constant  Value=B  VectorParams1D=off
  Sum : Sum  Inputs=|+++
  zdot : Outport
  wires:
  MatrizesA8/1 -> Matrix Multiply8/1
  Constant1/1 -> Matrix Multiply1/1
  z/1 -> Matrix Multiply3/2
  Matrix Multiply3/1 -> Sum/2
  Constant/1 -> Matrix Multiply3/1
  Matrix Multiply8/1 -> Matrix Multiply1/2
  Matrix Multiply1/1 -> Sum/1
  u/1 -> Matrix Multiply8/2
  Sum/1 -> zdot/1
  Constant2/1 -> Matrix Multiply2/1
  Matrix Multiply2/1 -> Sum/3
  y/1 -> Matrix Multiply2/2

== system bObserver/ROSMO_ROSLSO/Bank of ROSLSO/ROSLSO 2 Subsystems1/Reduced Order Derivate Z1 ==
  u : Inport
  y : Inport  Port=2
  z : Inport  Port=3
  Constant : Constant  Value=F  VectorParams1D=off
  Constant1 : Constant  Value=T  VectorParams1D=off
  Constant2 : Constant  Value=L  VectorParams1D=off
  Matrix Multiply{1..3,8} (4 alike) : Product  Multiplication=Matrix(*)
  MatrizesA8 : Constant  Value=B  VectorParams1D=off
  Sum : Sum  Inputs=|+++
  zdot : Outport
  wires:
  MatrizesA8/1 -> Matrix Multiply8/1
  Constant1/1 -> Matrix Multiply1/1
  z/1 -> Matrix Multiply3/2
  Matrix Multiply3/1 -> Sum/2
  Constant/1 -> Matrix Multiply3/1
  Matrix Multiply8/1 -> Matrix Multiply1/2
  Matrix Multiply1/1 -> Sum/1
  u/1 -> Matrix Multiply8/2
  Sum/1 -> zdot/1
  Constant2/1 -> Matrix Multiply2/1
  Matrix Multiply2/1 -> Sum/3
  y/1 -> Matrix Multiply2/2

== system bObserver/ROSMO_ROSLSO/Boost Converter Circuit/DC Source/Variable DC Source ==
  Vinput : Inport
  VinputAdd : Inport  Port=2
  VinputRemove : Inport  Port=3
  S3 : powerlib/Power Electronics/Ideal Switch  Ron=0.0000001  Lon=0  IC=0  Rs=1e8  Cs=inf  Measurements=on
  S5 : powerlib/Power Electronics/Ideal Switch  Ron=0.0000001  Lon=0  IC=0  Rs=1e8  Cs=inf  Measurements=on
  S7 : powerlib/Power Electronics/Ideal Switch  Ron=0.0000001  Lon=0  IC=0  Rs=1e8  Cs=inf  Measurements=on
  Terminator2 : Terminator
  Terminator3 : Terminator
  Terminator4 : Terminator
  u : powerlib/Electrical Sources/DC Voltage Source  Amplitude=u  Measurements=None
  u1 : powerlib/Electrical Sources/DC Voltage Source  Amplitude=uAdd  Measurements=None
  u2 : powerlib/Electrical Sources/DC Voltage Source  Amplitude=u  Measurements=None
  u3 : powerlib/Electrical Sources/DC Voltage Source  Amplitude=uRemove  Measurements=None
  u4 : powerlib/Electrical Sources/DC Voltage Source  Amplitude=u  Measurements=None
  V+ : PMIOPort  Side=Right
  V- : PMIOPort  Port=2  Side=Right
  wires:
  S5/1 -> Terminator4/1
  S7/1 -> Terminator2/1
  S3/1 -> Terminator3/1
  Vinput/1 -> S5/1
  VinputAdd/1 -> S3/1
  VinputRemove/1 -> S7/1
  connections:
  u1/LConn1 -- u2/RConn1
  u/LConn1 -- V-/RConn1 -- u4/LConn1 -- u2/LConn1
  S5/LConn1 -- V+/RConn1 -- S7/LConn1 -- S3/LConn1
  u3/RConn1 -- u4/RConn1
  u3/LConn1 -- S7/RConn1
  S3/RConn1 -- u1/RConn1
  u/RConn1 -- S5/RConn1

== system bObserver/ROSMO_ROSLSO/Boost Converter Circuit/Output Resistance/Subsystem ==
  RserieInput : Inport
  Rparallelinput : Inport  Port=2
  Ro : powerlib/Elements/Series RLC Branch  LConnTagsString=__new0  RConnTagsString=__new0  BranchType=R  Resistance=Ro  Inductance=1e-3  SetiL0=off  InitialCurrent=0  Capacitance=1e-6  Setx0=off  InitialVoltage=0  Measurements=None
  Rparallel : powerlib/Elements/Series RLC Branch  LConnTagsString=__new0  RConnTagsString=__new0  BranchType=R  Resistance=LoadRemoveResistor  Inductance=1e-3  SetiL0=off  InitialCurrent=0  Capacitance=1e-6  Setx0=off  InitialVoltage=0  Measurements=None
  Rserie : powerlib/Elements/Series RLC Branch  LConnTagsString=__new0  RConnTagsString=__new0  BranchType=R  Resistance=LoadAddResistor  Inductance=1e-3  SetiL0=off  InitialCurrent=0  Capacitance=1e-6  Setx0=off  InitialVoltage=0  Measurements=None
  S1 : powerlib/Power Electronics/Ideal Switch  Ron=0.0000001  Lon=0  IC=0  Rs=1e8  Cs=inf  Measurements=on
  S6 : powerlib/Power Electronics/Ideal Switch  Ron=0.0000001  Lon=0  IC=0  Rs=1e8  Cs=inf  Measurements=on
  Terminator5 : Terminator
  Terminator6 : Terminator
  Ro+ : PMIOPort  Side=Right
  Ro- : PMIOPort  Port=2  Side=Right
  wires:
  S6/1 -> Terminator6/1
  RserieInput/1 -> S1/1
  S1/1 -> Terminator5/1
  Rparallelinput/1 -> S6/1
  connections:
  Ro/RConn1 -- S1/LConn1 -- Rserie/RConn1 -- Rparallel/LConn1
  Ro/LConn1 -- Ro+/RConn1 -- S6/LConn1
  Rparallel/RConn1 -- S6/RConn1
  S1/RConn1 -- Ro-/RConn1 -- Rserie/LConn1

== system bObserver/ROSMO_ROSLSO/Fault Identification/Pattern Recognition Neural Network1/Layer 1 ==
  "p{1}" : Inport  PortDimensions=3
      mask Display: e = 0.06;c1 = [120 230 180]/255;c2 = ([120 230 180]+0)/(256+128);c3 = ([120 230 180]+128)/(256+128);patch([0 1 1 0],[0 0 1 1],c1);patch([0 1 1 1-e 1-e 0+e],[0 0 1 1-e 0+e 0+e],c2);patch([0 0 1 1-e 0+e 0+e],[0 1 1 1-e 1-e 0+e],c3);plot([0 1 1 0 0],[0 0 1 1 0]);
  Delays 1 : Subsystem
      mask Display: e = 0.06;c1 = [120 150 230]/255;c2 = ([120 150 230]+0)/383;c3 = ([120 150 230]+128)/383;patch([0 1 1 0],[0 0 1 1],c1);patch([0 1 1 1-e 1-e 0+e],[0 0 1 1-e 0+e 0+e],c2);patch([0 0 1 1-e 0+e 0+e],[0 1 1 1-e 1-e 0+e],c3);plot([0 1 1 0 0],[0 0 1 1 0]);disp('0');
  "IW{1,1}" : Subsystem
      mask Display: e = 0.06;c1 = [120 150 230]/255;c2 = ([120 150 230]+0)/383;c3 = ([120 150 230]+128)/383;patch([0 1 1 0],[0 0 1 1],c1);patch([0 1 1 1-e 1-e 0+e],[0 0 1 1-e 0+e 0+e],c2);patch([0 0 1 1-e 0+e 0+e],[0 1 1 1-e 1-e 0+e],c3);plot([0 1 1 0 0],[0 0 1 1 0]);disp('W');
  "b{1}" : Constant  Value=[-3.0907169643136906955760423443280160427093505859375;-8.5532408660313894444016113993711769580841064453125;26.179031484954197850356649723835289478302001953125;0.130591451617109999272514642143505625426769256591796875]
      mask Display: e = 0.06;c1 = [120 150 230]/255;c2 = ([120 150 230]+0)/383;c3 = ([120 150 230]+128)/383;patch([0 1 1 0],[0 0 1 1],c1);patch([0 1 1 1-e 1-e 0+e],[0 0 1 1-e 0+e 0+e],c2);patch([0 0 1 1-e 0+e 0+e],[0 1 1 1-e 1-e 0+e],c3);plot([0 1 1 0 0],[0 0 1 1 0]);disp('b');
  netsum : Sum  Inputs=2  InputSameDT=on  SaturateOnIntegerOverflow=on  OutDataTypeStr=Inherit: Same as first input
      mask Display: e = 0.06;c1 = [120 150 230]/255;c2 = ([120 150 230]+0)/383;c3 = ([120 150 230]+128)/383;patch([0 1 1 0],[0 0 1 1],c1);patch([0 1 1 1-e 1-e 0+e],[0 0 1 1-e 0+e 0+e],c2);patch([0 0 1 1-e 0+e 0+e],[0 1 1 1-e 1-e 0+e],c3);plot([0 1 1 0 0],[0 0 1 1 0]);disp('+');
  tansig : neural/Transfer Functions/tansig
  "a{1}" : Outport  InitialOutput=[0;0;0;0]
      mask Display: e = 0.06;c1 = [120 230 180]/255;c2 = ([120 230 180]+0)/(256+128);c3 = ([120 230 180]+128)/(256+128);patch([0 1 1 0],[0 0 1 1],c1);patch([0 1 1 1-e 1-e 0+e],[0 0 1 1-e 0+e 0+e],c2);patch([0 0 1 1-e 0+e 0+e],[0 1 1 1-e 1-e 0+e],c3);plot([0 1 1 0 0],[0 0 1 1 0]);
  wires:
  "p{1}"/1 -> Delays 1/1("p{1}")
  Delays 1/1("pd{1,1}") -> "IW{1,1}"/1("pd{1,1}")
  "IW{1,1}"/1("iz{1,1}") -> netsum/1
  "b{1}"/1 -> netsum/2
  netsum/1 -> tansig/1
  tansig/1 -> "a{1}"/1

== system bObserver/ROSMO_ROSLSO/Fault Identification/Pattern Recognition Neural Network1/Layer 2 ==
  "a{1} " : Inport  PortDimensions=4
      mask Display: e = 0.06;c1 = [120 230 180]/255;c2 = ([120 230 180]+0)/(256+128);c3 = ([120 230 180]+128)/(256+128);patch([0 1 1 0],[0 0 1 1],c1);patch([0 1 1 1-e 1-e 0+e],[0 0 1 1-e 0+e 0+e],c2);patch([0 0 1 1-e 0+e 0+e],[0 1 1 1-e 1-e 0+e],c3);plot([0 1 1 0 0],[0 0 1 1 0]);
  Delays 1 : Subsystem
      mask Display: e = 0.06;c1 = [120 150 230]/255;c2 = ([120 150 230]+0)/383;c3 = ([120 150 230]+128)/383;patch([0 1 1 0],[0 0 1 1],c1);patch([0 1 1 1-e 1-e 0+e],[0 0 1 1-e 0+e 0+e],c2);patch([0 0 1 1-e 0+e 0+e],[0 1 1 1-e 1-e 0+e],c3);plot([0 1 1 0 0],[0 0 1 1 0]);disp('0');
  "LW{2,1}" : Subsystem
      mask Display: e = 0.06;c1 = [120 150 230]/255;c2 = ([120 150 230]+0)/383;c3 = ([120 150 230]+128)/383;patch([0 1 1 0],[0 0 1 1],c1);patch([0 1 1 1-e 1-e 0+e],[0 0 1 1-e 0+e 0+e],c2);patch([0 0 1 1-e 0+e 0+e],[0 1 1 1-e 1-e 0+e],c3);plot([0 1 1 0 0],[0 0 1 1 0]);disp('W');
  "b{2}" : Constant  Value=[-2.302427575546979188203522426192648708820343017578125;-5.91134493996858534359262193902395665645599365234375;6.8980698616354221286428582970984280109405517578125;0.77959090259712271464564992129453457891941070556640625;-0.782333279931369585113998255110345780849456787109375]
      mask Display: e = 0.06;c1 = [120 150 230]/255;c2 = ([120 150 230]+0)/383;c3 = ([120 150 230]+128)/383;patch([0 1 1 0],[0 0 1 1],c1);patch([0 1 1 1-e 1-e 0+e],[0 0 1 1-e 0+e 0+e],c2);patch([0 0 1 1-e 0+e 0+e],[0 1 1 1-e 1-e 0+e],c3);plot([0 1 1 0 0],[0 0 1 1 0]);disp('b');
  netsum : Sum  Inputs=2  InputSameDT=on  SaturateOnIntegerOverflow=on  OutDataTypeStr=Inherit: Same as first input
      mask Display: e = 0.06;c1 = [120 150 230]/255;c2 = ([120 150 230]+0)/383;c3 = ([120 150 230]+128)/383;patch([0 1 1 0],[0 0 1 1],c1);patch([0 1 1 1-e 1-e 0+e],[0 0 1 1-e 0+e 0+e],c2);patch([0 0 1 1-e 0+e 0+e],[0 1 1 1-e 1-e 0+e],c3);plot([0 1 1 0 0],[0 0 1 1 0]);disp('+');
  softmax : neural/Transfer Functions/softmax
      settings: SourceProductBaseCode=NN
  "a{2}" : Outport  InitialOutput=[0;0;0;0;0]
      mask Display: e = 0.06;c1 = [120 230 180]/255;c2 = ([120 230 180]+0)/(256+128);c3 = ([120 230 180]+128)/(256+128);patch([0 1 1 0],[0 0 1 1],c1);patch([0 1 1 1-e 1-e 0+e],[0 0 1 1-e 0+e 0+e],c2);patch([0 0 1 1-e 0+e 0+e],[0 1 1 1-e 1-e 0+e],c3);plot([0 1 1 0 0],[0 0 1 1 0]);
  wires:
  "a{1} "/1 -> Delays 1/1("p{2}")
  Delays 1/1("pd{2,1}") -> "LW{2,1}"/1("ad{2,1}")
  "LW{2,1}"/1("lz{2,1}") -> netsum/1
  "b{2}"/1 -> netsum/2
  netsum/1 -> softmax/1
  softmax/1 -> "a{2}"/1

== system bObserver/ROSMO_ROSLSO/Fault Identification/Pattern Recognition Neural Network1/Process Input 1 ==
  x : Inport  PortDimensions=3
      mask Display: e = 0.06;c1 = [120 230 180]/255;c2 = ([120 230 180]+0)/(256+128);c3 = ([120 230 180]+128)/(256+128);patch([0 1 1 0],[0 0 1 1],c1);patch([0 1 1 1-e 1-e 0+e],[0 0 1 1-e 0+e 0+e],c2);patch([0 0 1 1-e 0+e 0+e],[0 1 1 1-e 1-e 0+e],c3);plot([0 1 1 0 0],[0 0 1 1 0]);
  mapminmax : neural/Processing Functions/mapminmax  xmin=[0;0;-2641.94920061935135890962556005]  xmax=[786.388396902503131968842353672;8926.40391005816127290017902851;8647.99703455211783875711262226]  ymin=-1  ymax=1
  p : Outport  PortDimensions=3
      mask Display: e = 0.06;c1 = [120 230 180]/255;c2 = ([120 230 180]+0)/(256+128);c3 = ([120 230 180]+128)/(256+128);patch([0 1 1 0],[0 0 1 1],c1);patch([0 1 1 1-e 1-e 0+e],[0 0 1 1-e 0+e 0+e],c2);patch([0 0 1 1-e 0+e 0+e],[0 1 1 1-e 1-e 0+e],c3);plot([0 1 1 0 0],[0 0 1 1 0]);
  wires:
  x/1 -> mapminmax/1
  mapminmax/1 -> p/1

== system bObserver/ROSMO_ROSLSO/Fault Identification/Pattern Recognition Neural Network1/Process Output 1 ==
  a : Inport  PortDimensions=5
      mask Display: e = 0.06;c1 = [120 230 180]/255;c2 = ([120 230 180]+0)/(256+128);c3 = ([120 230 180]+128)/(256+128);patch([0 1 1 0],[0 0 1 1],c1);patch([0 1 1 1-e 1-e 0+e],[0 0 1 1-e 0+e 0+e],c2);patch([0 0 1 1-e 0+e 0+e],[0 1 1 1-e 1-e 0+e],c3);plot([0 1 1 0 0],[0 0 1 1 0]);
  y : Outport  PortDimensions=5
      mask Display: e = 0.06;c1 = [120 230 180]/255;c2 = ([120 230 180]+0)/(256+128);c3 = ([120 230 180]+128)/(256+128);patch([0 1 1 0],[0 0 1 1],c1);patch([0 1 1 1-e 1-e 0+e],[0 0 1 1-e 0+e 0+e],c2);patch([0 0 1 1-e 0+e 0+e],[0 1 1 1-e 1-e 0+e],c3);plot([0 1 1 0 0],[0 0 1 1 0]);
  wires:
  a/1 -> y/1

== system bObserver/ROSMO_ROSLSO/SMO/ErrorGenerator/If Action Subsystem ==
  e_y : Inport
  Action Port : ActionPort  ActionPortLabel=if(u1 ~= 0)
  Matrix Multiply : Product  Multiplication=Matrix(*)
  Matrix Multiply1 : Product
  Matrizes A1 : Constant  Value=rho
  Matrizes A2 : Constant  Value=F  VectorParams1D=off
  Normalization : dspmathops/Normalization  NormType=2-norm  Bias=1e-10  NormOver=Each column  Dimension=1  roundingMode=Floor  overflowMode=off  accumDataTypeStr=Inherit: Same as product output  accumLastDataTypeStr=Inherit: Same as product output  outputDataTypeStr=Inherit: Same as product output  outputMin=[]  outputMax=[]  outputLastDataTypeStr=Inherit: Same as product output
  v : Outport
  wires:
  Matrix Multiply/1 -> Normalization/1
  Matrizes A2/1 -> Matrix Multiply/1
  Normalization/1 -> Matrix Multiply1/2
  e_y/1 -> Matrix Multiply/2
  Matrizes A1/1 -> Matrix Multiply1/1
  Matrix Multiply1/1 -> v/1

== system bObserver/ROSMO_ROSLSO/SMO/ErrorGenerator/If Action Subsystem1 ==
  e_y : Inport
  Action Port : ActionPort  ActionPortLabel=else
  v : Outport
  wires:
  e_y/1 -> v/1

== system bObserver/ROSMO_ROSLSO/SMO/Sliding Mode Observer 5/ObserverDynamics ==
  ey : Inport
  v : Inport  Port=2
  sigma : Inport  Port=3
  Gain : Gain  Gain=Atilde1  Multiplication=Matrix(K*u)
  Gain1 : Gain  Gain=G  Multiplication=Matrix(K*u)
  Gain3 : Gain  Gain=Dtilde1  Multiplication=Matrix(K*u)
  Gain5 : Gain  Gain=Atilde2  Multiplication=Matrix(K*u)
  Gain7 : Gain  Gain=Dtilde2  Multiplication=Matrix(K*u)
  Integral : Subsystem
  Sum : Sum  Inputs=|+++
  Sum1 : Sum  Inputs=|+++
  Switch1 : Switch  Criteria=u2 > Threshold
  e_tilde_hat : Outport
  wires:
  sigma/1 -> Switch1/2
  Switch1/1 -> Integral/1(e_hat_dot)  "v"
  Integral/1(e_hat) -> Gain/1, e_tilde_hat/1, Gain5/1
  ey/1 -> Gain1/1
  v/1 -> Gain7/1, Gain3/1
  Sum1/1 -> Switch1/3
  Sum/1 -> Switch1/1
  Gain7/1 -> Sum1/2
  Gain5/1 -> Sum1/3
  Gain3/1 -> Sum/1
  Gain1/1 -> Sum1/1, Sum/2
  Gain/1 -> Sum/3

== system bObserver/Slding Mode/Boost Converter/TipoEntrada/disturbio ==
  Step1 : Step  SampleTime=0
  Step2 : Step  Time=1.1  After=-1  SampleTime=0
  Sum : Sum  Inputs=|++
  disturbio : Outport
  wires:
  Sum/1 -> disturbio/1
  Step2/1 -> Sum/2
  Step1/1 -> Sum/1

== system bObserver/Slding Mode/Boost Converter/TipoEntrada/disturbio1 ==
  Step1 : Step  Time=1.2  SampleTime=0
  Step2 : Step  Time=1.4  After=-1  SampleTime=0
  Sum : Sum  Inputs=|++
  disturbio : Outport
  wires:
  Sum/1 -> disturbio/1
  Step2/1 -> Sum/2
  Step1/1 -> Sum/1

== system bObserver/Slding Mode/Boost Converter/TipoEntrada/disturbio2 ==
  Step1 : Step  Time=1.2  SampleTime=0
  Step2 : Step  Time=1.4  After=-1  SampleTime=0
  Sum : Sum  Inputs=|++
  disturbio : Outport
  wires:
  Sum/1 -> disturbio/1
  Step2/1 -> Sum/2
  Step1/1 -> Sum/1

== system bObserver/Slding Mode/Boost Converter/TipoEntrada/disturbio3 ==
  Step1 : Step  SampleTime=0
  Step2 : Step  Time=1.1  After=-1  SampleTime=0
  Sum : Sum  Inputs=|++
  disturbio : Outport
  wires:
  Sum/1 -> disturbio/1
  Step2/1 -> Sum/2
  Step1/1 -> Sum/1

== system bObserver/Slding Mode/Controlador1/SlidingSurface/If Action Subsystem ==
  S : Inport
  Action Port : ActionPort  ActionPortLabel=if(u1 ~= 0)
  Sign : Signum
  d : Outport
  wires:
  S/1 -> Sign/1
  Sign/1 -> d/1

== system bObserver/Slding Mode/Controlador1/SlidingSurface/If Action Subsystem2 ==
  S : Inport
  ep : Inport  Port=2
  Action Port : ActionPort  ActionPortLabel=else
  Divide : Product  Inputs=*/
  d : Outport
  wires:
  S/1 -> Divide/1
  ep/1 -> Divide/2
  Divide/1 -> d/1
